simulink model "SIM_nonlinear_LQR_dis"  (R2023a)
settings: Solver=ode23t  StartTime=0.0  StopTime=30  MaxStep=1e-4  RelTol=1e-3
values from neighbouring files (symbols this model uses):
  input_dis = 0    [param.m]
  input_dis_time = 10    [param.m]
  Kr = sqrt(Q(1, 1)/R)    [param.m]
undefined symbols (not defined in the file or in its folder): K
libraries: dspsrcs4 x3
settings Model: Creator=edzel  LastModifiedBy=edzel

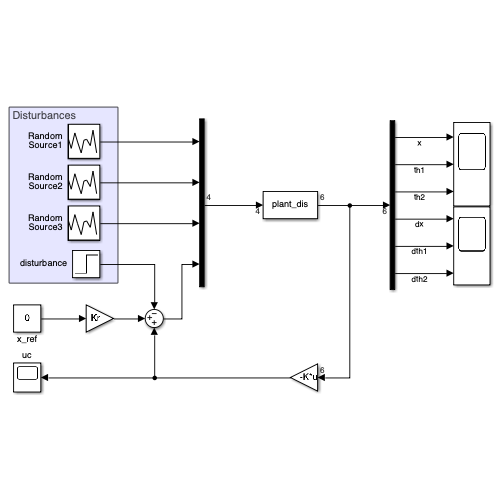
[thumbnail: Simulink's stored preview of the top-level diagram]
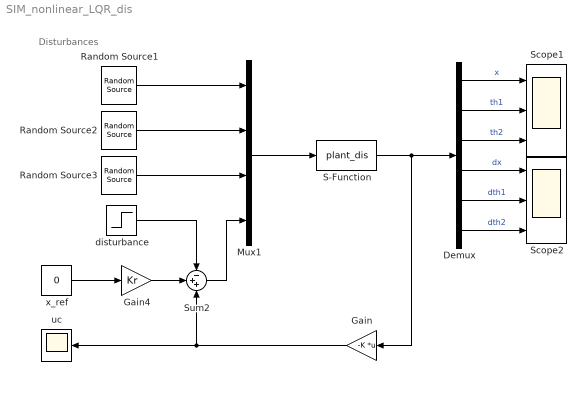
== system SIM_nonlinear_LQR_dis ==
  note: Disturbances
  Demux : Demux  Outputs=6
  Gain : Gain  Gain=-K  Multiplication=Matrix(K*u)
  Gain4 : Gain  Gain=Kr
  Mux1 : Mux
  Random Source1 : dspsrcs4/Random Source  SrcType=Gaussian  NormMethod=Ziggurat  CltLength=12  MinVal=0  MaxVal=1  MeanVal=d1_mean  VarVal=d1_variance  RepMode=Specify seed  rawSeed=42  IsInherit=off  SampMode=Continuous  SampTime=1  SampFrame=1  DataType=Double  OutComplex=Real  OutputFrames=off
  Random Source2 : dspsrcs4/Random Source  SrcType=Gaussian  NormMethod=Ziggurat  CltLength=12  MinVal=0  MaxVal=1  MeanVal=d2_mean  VarVal=d2_variance  RepMode=Specify seed  rawSeed=42  IsInherit=off  SampMode=Continuous  SampTime=1  SampFrame=1  DataType=Double  OutComplex=Real  OutputFrames=off
  Random Source3 : dspsrcs4/Random Source  SrcType=Gaussian  NormMethod=Ziggurat  CltLength=12  MinVal=0  MaxVal=1  MeanVal=d3_mean  VarVal=d3_variance  RepMode=Specify seed  rawSeed=42  IsInherit=off  SampMode=Continuous  SampTime=1  SampFrame=1  DataType=Double  OutComplex=Real  OutputFrames=off
  S-Function : S-Function  FunctionName=plant_dis  Parameters=CoeF1, CoeF2, CoeF3, theta1_rad, theta2_rad  SFunctionDeploymentMode=off  EnableBusSupport=off
  Scope1 : Scope  NumInputPorts=3
  Scope2 : Scope  NumInputPorts=3
  Sum2 : Sum  Inputs=-++
  disturbance : Step  Time=input_dis_time  After=input_dis  SampleTime=0
  uc : Scope
  x_ref : Constant  Value=0
  wires:
  x_ref/1 -> Gain4/1
  Gain4/1 -> Sum2/2
  Gain/1 -> Sum2/3, uc/1
  disturbance/1 -> Sum2/1
  Random Source3/1 -> Mux1/3
  Random Source2/1 -> Mux1/2
  Random Source1/1 -> Mux1/1
  Mux1/1 -> S-Function/1
  Sum2/1 -> Mux1/4
  S-Function/1 -> Demux/1, Gain/1
  Demux/4 -> Scope2/1  "dx"
  Demux/3 -> Scope1/3  "th2"
  Demux/5 -> Scope2/2  "dth1"
  Demux/6 -> Scope2/3  "dth2"
  Demux/2 -> Scope1/2  "th1"
  Demux/1 -> Scope1/1  "x"
